simulink model "model_quad"  (R2013b)
settings: Solver=ode23  StartTime=0.0  StopTime=30  RelTol=1e-3
values from neighbouring files (symbols this model uses):
  b = 3.25*10^(-5)    (= 3.25e-05)    [const_global.m]    (also in quadvar.m)
  g = 10    [const_global.m]    (also in quadvar.m = 9.81)
  m = 0.65    [const_global.m]    (also in quadvar.m)
settings Model: Creator=Ardy Seto Priambodo  LastModifiedBy=asd
settings SolverCC: MaxConsecutiveMinStep=10000
settings DataIOCC: SignalLoggingSaveFormat=ModelDataLogs
settings OptimizationCC: ExpressionDepthLimit=2147483647
settings DebuggingCC: FcnCallInpInsideContextMsg=UseLocalSettings  StateNameClashWarn=warning
settings GRTTargetCC: CombineOutputUpdateFcns=off  GRTInterface=on

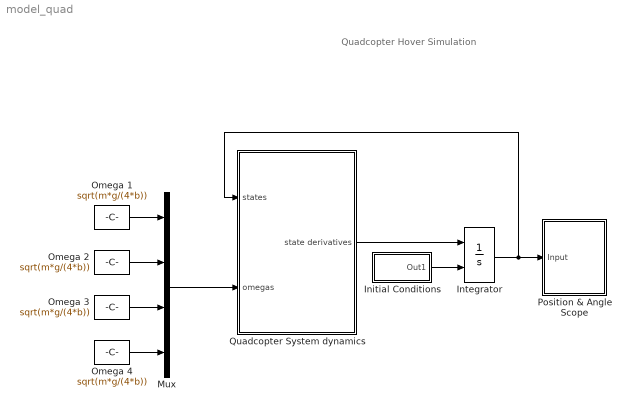
== system model_quad ==
  note: Quadcopter
      | Hover Simulation
  Initial Conditions : Subsystem
  Integrator : Integrator  InitialConditionSource=external
  Mux : Mux
  Omega {1..4} (4 alike) : Constant  Value=sqrt(m*g/(4*b))
  Position & Angle Scope : Subsystem
  Quadcopter System dynamics : Subsystem
  wires:
  Omega 1/1 -> Mux/1
  Omega 2/1 -> Mux/2
  Omega 3/1 -> Mux/3
  Omega 4/1 -> Mux/4
  Mux/1 -> Quadcopter System dynamics/2(omegas)
  Initial Conditions/1(Out1) -> Integrator/2
  Quadcopter System dynamics/1(state derivatives) -> Integrator/1
  Integrator/1 -> Position & Angle Scope/1(Input), Quadcopter System dynamics/1(states)

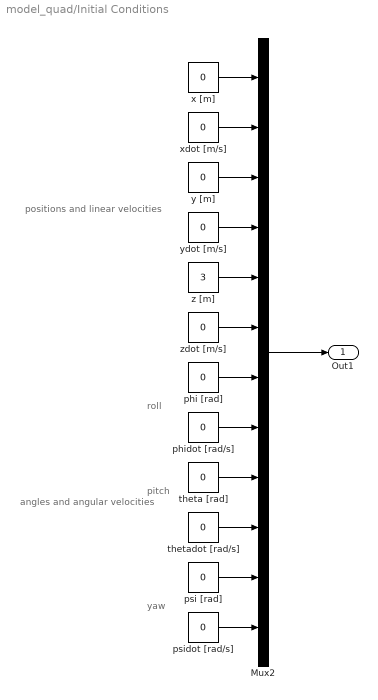
== system model_quad/Initial Conditions ==
  note: positions and linear velocities
  note: angles and angular velocities
  note: yaw
  note: pitch
  note: roll
  Mux2 : Mux  Inputs=12
  phi [rad] : Constant  Value=0
  phidot [rad/s] : Constant  Value=0
  psi [rad] : Constant  Value=0
  psidot [rad/s] : Constant  Value=0
  theta [rad] : Constant  Value=0
  thetadot [rad/s] : Constant  Value=0
  x [m] : Constant  Value=0
  xdot [m/s] : Constant  Value=0
  y [m] : Constant  Value=0
  ydot [m/s] : Constant  Value=0
  z [m] : Constant  Value=3
  zdot [m/s] : Constant  Value=0
  Out1 : Outport
  wires:
  x [m]/1 -> Mux2/1
  xdot [m/s]/1 -> Mux2/2
  y [m]/1 -> Mux2/3
  ydot [m/s]/1 -> Mux2/4
  z [m]/1 -> Mux2/5
  zdot [m/s]/1 -> Mux2/6
  phi [rad]/1 -> Mux2/7
  phidot [rad/s]/1 -> Mux2/8
  theta [rad]/1 -> Mux2/9
  thetadot [rad/s]/1 -> Mux2/10
  psi [rad]/1 -> Mux2/11
  psidot [rad/s]/1 -> Mux2/12
  Mux2/1 -> Out1/1

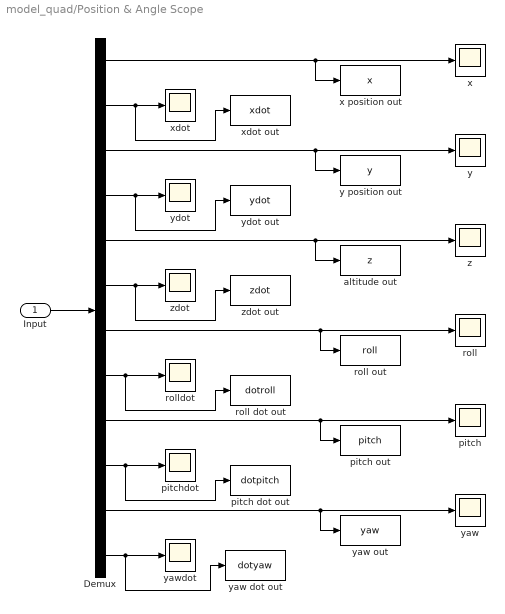
== system model_quad/Position & Angle Scope ==
  Input : Inport
  Demux : Demux  Outputs=12
  altitude out : ToWorkspace  VariableName=z  SampleTime=-1
  pitch : Scope
      settings: TimeRange=4  YMin=-0.055  YMax=0.045
  pitch dot out : ToWorkspace  VariableName=dotpitch  SampleTime=-1
  pitch out : ToWorkspace  VariableName=pitch  SampleTime=-1
  pitchdot : Scope
      settings: YMin=-1.75  YMax=1.75  SaveName=ScopeData4
  roll : Scope
      settings: TimeRange=0.25  YMin=-0.031  YMax=-0.008
  roll dot out : ToWorkspace  VariableName=dotroll  SampleTime=-1
  roll out : ToWorkspace  VariableName=roll  SampleTime=-1
  rolldot : Scope
      settings: TimeRange=7  YMin=-0.15  YMax=0.125  SaveName=ScopeData5
  x : Scope
      settings: TimeRange=20  YMin=-0.5  YMax=2.5  SaveName=ScopeData6
  x position out : ToWorkspace  VariableName=x  SampleTime=-1
  xdot : Scope
      settings: TimeRange=5  YMin=-4.75e-015  YMax=0  SaveName=ScopeData7
  xdot out : ToWorkspace  VariableName=xdot  SampleTime=-1
  y : Scope
      settings: TimeRange=5  YMin=1.825  YMax=2.075  SaveName=ScopeData8
  y position out : ToWorkspace  VariableName=y  SampleTime=-1
  yaw : Scope
      settings: TimeRange=5  YMin=-0.02  YMax=0.0125  SaveName=ScopeData2
  yaw dot out : ToWorkspace  VariableName=dotyaw  SampleTime=-1
  yaw out : ToWorkspace  VariableName=yaw  SampleTime=-1
  yawdot : Scope
      settings: TimeRange=18  YMin=-0.275  YMax=0.15  SaveName=ScopeData9
  ydot : Scope
      settings: TimeRange=5  YMin=-143.75  YMax=-141.75  SaveName=ScopeData10
  ydot out : ToWorkspace  VariableName=ydot  SampleTime=-1
  z : Scope
      settings: TimeRange=5  YMin=2.9255  YMax=2.935  SaveName=ScopeData11
  zdot : Scope
      settings: TimeRange=10  YMin=-110.5  YMax=-107.25  SaveName=ScopeData12
  zdot out : ToWorkspace  VariableName=zdot  SampleTime=-1
  wires:
  Input/1 -> Demux/1
  Demux/2 -> xdot/1, xdot out/1
  Demux/4 -> ydot/1, ydot out/1
  Demux/6 -> zdot/1, zdot out/1
  Demux/1 -> x position out/1, x/1
  Demux/3 -> y position out/1, y/1
  Demux/5 -> altitude out/1, z/1
  Demux/8 -> rolldot/1, roll dot out/1
  Demux/10 -> pitchdot/1, pitch dot out/1
  Demux/12 -> yawdot/1, yaw dot out/1
  Demux/7 -> roll/1, roll out/1
  Demux/9 -> pitch/1, pitch out/1
  Demux/11 -> yaw/1, yaw out/1

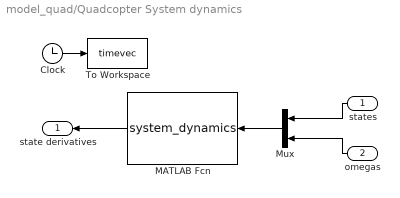
== system model_quad/Quadcopter System dynamics ==
  states : Inport
  omegas : Inport  Port=2
  Clock : Clock
  MATLAB Fcn : MATLABFcn  MATLABFcn=system_dynamics  OutputDimensions=12
  Mux : Mux  Inputs=2
  To Workspace : ToWorkspace  VariableName=timevec  SampleTime=-1
  state derivatives : Outport
  wires:
  Mux/1 -> MATLAB Fcn/1
  MATLAB Fcn/1 -> state derivatives/1
  omegas/1 -> Mux/2
  states/1 -> Mux/1
  Clock/1 -> To Workspace/1
